simulink model "XfmrProtection_300MVA_Yd1"  (R2023a)
settings: Solver=ode23tb  StartTime=0.0  StopTime=0.30  MaxStep=2e-5  RelTol=1e-5
libraries: spsThreePhaseFaultLib x5, spsThreePhaseSeriesRLCBranchLib x5, spsThreePhaseVIMeasurementLib x4, spsThreePhaseBreakerLib x1, spsGroundLib x1, spsThreePhaseTransformerTwoWindingsLib x1, spsThreePhaseSourceLib x1, spspowerguiLib x1
settings Model: Creator=Abeer  LastModifiedBy=Abeer

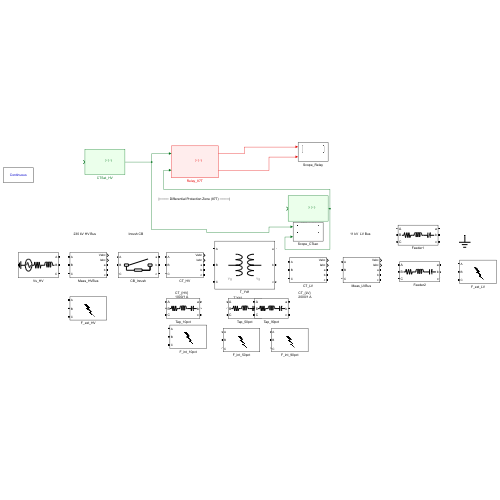
[thumbnail: Simulink's stored preview of the top-level diagram]
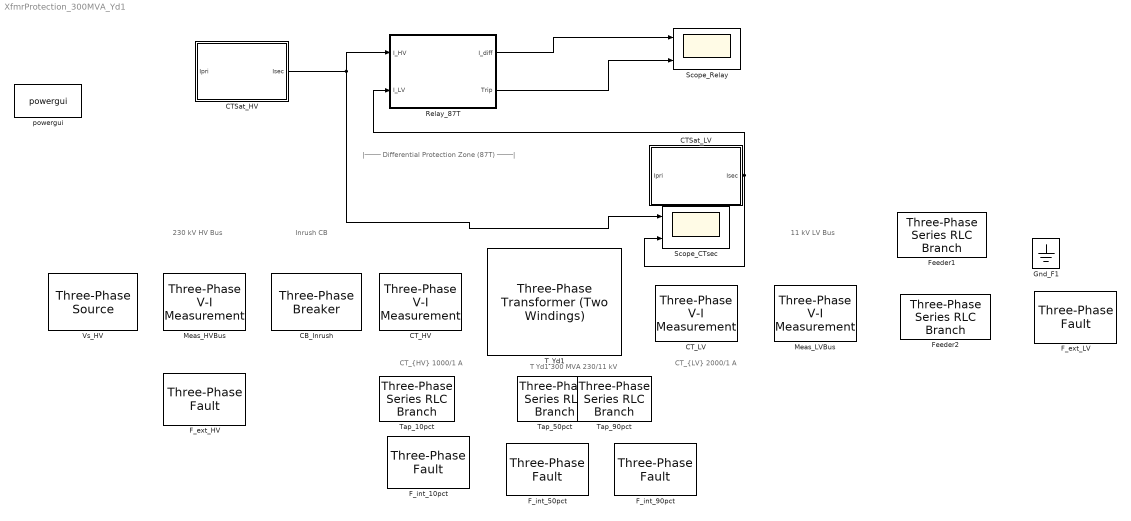
== system XfmrProtection_300MVA_Yd1 ==
  note: 230 kV HV Bus
  note: 11 kV LV Bus
  note: T Yd1
      | 300 MVA
      | 230/11 kV
  note: CT_{HV}
      | 1000/1 A
  note: CT_{LV}
      | 2000/1 A
  note: Inrush CB
  note: |──── Differential Protection Zone (87T) ────|
  CB_Inrush : spsThreePhaseBreakerLib/Three-Phase Breaker  InitialState=open  SwitchA=on  SwitchB=on  SwitchC=on  SwitchTimes="[1/60  5/60]"  External=off  BreakerResistance=0.01  SnubberResistance=1e6  SnubberCapacitance=inf  Measurements=None
  CTSat_HV : Subsystem
      mask Display: color([0 0.45 0.1]);patch([0.08 0.92 0.92 0.08],[0.08 0.08 0.92 0.92],[0.92 1.0 0.92]);text(0.5,0.62,'CTSat_HV','hor','center','FontSize',8,'FontWeight','bold');text(0.5,0.32,'Sat CT','hor','center','FontSize',7);text(0.5,0.15,'1/1000','hor','center','FontSize',7);
  CTSat_LV : Subsystem
      mask Display: color([0 0.45 0.1]);patch([0.08 0.92 0.92 0.08],[0.08 0.08 0.92 0.92],[0.92 1.0 0.92]);text(0.5,0.62,'CTSat_LV','hor','center','FontSize',8,'FontWeight','bold');text(0.5,0.32,'Sat CT','hor','center','FontSize',7);text(0.5,0.15,'1/2000','hor','center','FontSize',7);
  CT_HV : spsThreePhaseVIMeasurementLib/Three-Phase V-I Measurement  VoltageMeasurement=phase-to-ground  SetLabelV=off  LabelV=Vabc  Vpu=off  VpuLL=off  CurrentMeasurement=yes  SetLabelI=off  LabelI=Iabc  Ipu=off  Pbase=100e6  Vbase=500e3  OutputType=Complex  PhasorSimulation=off  PSBequivalent=0
  CT_LV : spsThreePhaseVIMeasurementLib/Three-Phase V-I Measurement  VoltageMeasurement=phase-to-ground  SetLabelV=off  LabelV=Vabc  Vpu=off  VpuLL=off  CurrentMeasurement=yes  SetLabelI=off  LabelI=Iabc  Ipu=off  Pbase=100e6  Vbase=500e3  OutputType=Complex  PhasorSimulation=off  PSBequivalent=0
  F_ext_HV : spsThreePhaseFaultLib/Three-Phase Fault  InitialStates=0  FaultA=on  FaultB=on  FaultC=on  GroundFault=on  SwitchTimes="[1/60  5/60]"  External=off  SwitchStatus=NaN  FaultResistance=0.001  GroundResistance=0.01  SnubberResistance=1e6  SnubberCapacitance=inf  Measurements=None
  F_ext_LV : spsThreePhaseFaultLib/Three-Phase Fault  InitialStates=0  FaultA=on  FaultB=on  FaultC=on  GroundFault=on  SwitchTimes="[1/60  5/60]"  External=off  SwitchStatus=NaN  FaultResistance=0.001  GroundResistance=0.01  SnubberResistance=1e6  SnubberCapacitance=inf  Measurements=None
  F_int_10pct : spsThreePhaseFaultLib/Three-Phase Fault  InitialStates=0  FaultA=on  FaultB=on  FaultC=on  GroundFault=on  SwitchTimes="[1/60  5/60]"  External=off  SwitchStatus=NaN  FaultResistance=0.001  GroundResistance=0.01  SnubberResistance=1e6  SnubberCapacitance=inf  Measurements=None
  F_int_50pct : spsThreePhaseFaultLib/Three-Phase Fault  InitialStates=0  FaultA=on  FaultB=on  FaultC=on  GroundFault=on  SwitchTimes="[1/60  5/60]"  External=off  SwitchStatus=NaN  FaultResistance=0.001  GroundResistance=0.01  SnubberResistance=1e6  SnubberCapacitance=inf  Measurements=None
  F_int_90pct : spsThreePhaseFaultLib/Three-Phase Fault  InitialStates=0  FaultA=on  FaultB=on  FaultC=on  GroundFault=on  SwitchTimes="[1/60  5/60]"  External=off  SwitchStatus=NaN  FaultResistance=0.001  GroundResistance=0.01  SnubberResistance=1e6  SnubberCapacitance=inf  Measurements=None
  Feeder1 : spsThreePhaseSeriesRLCBranchLib/Three-Phase Series RLC Branch  LConnTagsString=A|B|C  RConnTagsString=A|B|C  BranchType=RLC  Resistance=1  Inductance=1e-3  Capacitance=1e-6  Measurements=None
  Feeder2 : spsThreePhaseSeriesRLCBranchLib/Three-Phase Series RLC Branch  LConnTagsString=A|B|C  RConnTagsString=A|B|C  BranchType=RLC  Resistance=1  Inductance=1e-3  Capacitance=1e-6  Measurements=None
  Gnd_F1 : spsGroundLib/Ground  LConnTagsString=a
  Meas_HVBus : spsThreePhaseVIMeasurementLib/Three-Phase V-I Measurement  VoltageMeasurement=phase-to-ground  SetLabelV=off  LabelV=Vabc  Vpu=off  VpuLL=off  CurrentMeasurement=yes  SetLabelI=off  LabelI=Iabc  Ipu=off  Pbase=100e6  Vbase=500e3  OutputType=Complex  PhasorSimulation=off  PSBequivalent=0
  Meas_LVBus : spsThreePhaseVIMeasurementLib/Three-Phase V-I Measurement  VoltageMeasurement=phase-to-ground  SetLabelV=off  LabelV=Vabc  Vpu=off  VpuLL=off  CurrentMeasurement=yes  SetLabelI=off  LabelI=Iabc  Ipu=off  Pbase=100e6  Vbase=500e3  OutputType=Complex  PhasorSimulation=off  PSBequivalent=0
  Relay_87T : Subsystem
      mask Display: color('red');patch([0.05 0.95 0.95 0.05],[0.05 0.05 0.95 0.95],[1 0.93 0.93]);text(0.5,0.60,'87T','hor','center','ver','middle','FontSize',14,'FontWeight','bold');text(0.5,0.20,'Diff Relay','hor','center','FontSize',7);
  Scope_CTsec : Scope  NumInputPorts=2
  Scope_Relay : Scope  NumInputPorts=2
  T_Yd1 : spsThreePhaseTransformerTwoWindingsLib/Three-Phase Transformer (Two Windings)  Winding1Connection=Yg  Winding2Connection=Yg  CoreType=Three single-phase transformers  SetSaturation=off  Hysteresis=off  DataFile='hysteresis'  SetInitialFlux=off  Measurements=None  UNITS=pu  NominalPower=[ 250e6 , 60 ]  Winding1=[ 735e3 , 0.002 , 0.08 ]  Winding2=[ 315e3 , 0.002 , 0.08 ]  Rm=500  Lm=500  L0=0.5  Saturation=[ 0,0 ; 0.0024,1.2 ; 1.0,1.52 ]  InitialFluxes=[ 0.8 , -0.8 , 0.7 ]  BreakLoop=off  DiscreteSolver=Trapezoidal iterative  DataType=off  TransfoNumber=1
  Tap_10pct : spsThreePhaseSeriesRLCBranchLib/Three-Phase Series RLC Branch  LConnTagsString=A|B|C  RConnTagsString=A|B|C  BranchType=RLC  Resistance=1  Inductance=1e-3  Capacitance=1e-6  Measurements=None
  Tap_50pct : spsThreePhaseSeriesRLCBranchLib/Three-Phase Series RLC Branch  LConnTagsString=A|B|C  RConnTagsString=A|B|C  BranchType=RLC  Resistance=1  Inductance=1e-3  Capacitance=1e-6  Measurements=None
  Tap_90pct : spsThreePhaseSeriesRLCBranchLib/Three-Phase Series RLC Branch  LConnTagsString=A|B|C  RConnTagsString=A|B|C  BranchType=RLC  Resistance=1  Inductance=1e-3  Capacitance=1e-6  Measurements=None
  Vs_HV : spsThreePhaseSourceLib/Three-Phase Source  InternalConnection=Yg  VoltagePhases=off  Voltage=25e3  PhaseAngle=0  Voltage_phases=[25e3 25e3 25e3]/sqrt(3)  PhaseAngles_phases=[0 -120 +120]  Frequency=60  NonIdealSource=on  SpecifyImpedance=off  Resistance=0.8929  Inductance=16.58e-3  ShortCircuitLevel=100e6  BaseVoltage=25e3  XRratio=7  BusType=swing  Pref=10e3  Qref=0  Prefabc=[10e3, 10e3, 10e3]  Qrefabc=[0, 0, 0]  Qmin=-inf  Qmax=inf
  powergui : spspowerguiLib/powergui  Priority=1  SimulationMode=Continuous  SampleTime=50e-6  frequency=60  Iterations=50  frequencyindice=60  Pbase=100e6  ErrMax=1e-4  UnitsV=kV  UnitsW=MW  buscounter=0  FunctionMessages=off  echomessages=off  EnableUseOfTLC=off  CurrentSourceSwitches=off  DisableSnubberDevices=off  DisableRonSwitches=off  DisableVfSwitches=off  DisplayEquations=off  AutomaticDiscreteSolvers=off  SolverType=Tustin/Backward Euler (TBE)  Interpol=off  ExternalGateDelay=off  methode=off  Ts=100  x0status=blocks  SPID=on  SwTol=0  HookPort=off  NonlinearTolerance=1e-4  nMaxIteration=100  ContinueOnMaxIteration=off  RestoreLinks=warning  ResistiveCurrentMeasurement=off  Frange=[0:2:500]  Ylog=off  Xlog=on  ShowGrid=off  save=off  variable=ZData  structure=0  ZoomFFT=off  StartTime=0.0  cycles=1  DisplayStyle=1  fundamental=60  FreqAxis=off  MaxFrequency=1000  frequencyindicesteady=1  RmsSteady=1  display=off
  wires:
  CTSat_HV/1(Isec) -> Scope_CTsec/1, Relay_87T/1(I_HV)
  CTSat_LV/1(Isec) -> Relay_87T/2(I_LV), Scope_CTsec/2
  Relay_87T/1(I_diff) -> Scope_Relay/1
  Relay_87T/2(Trip) -> Scope_Relay/2

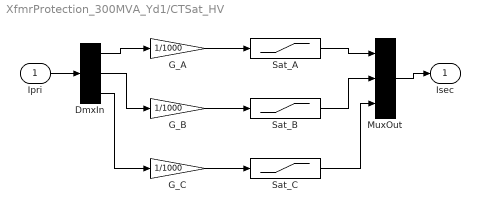
== system XfmrProtection_300MVA_Yd1/CTSat_HV ==
  Ipri : Inport
  DmxIn : Demux  Outputs=3
  G_A : Gain  Gain=1/1000
  G_B : Gain  Gain=1/1000
  G_C : Gain  Gain=1/1000
  MuxOut : Mux  Inputs=3
  Sat_A : Saturate  UpperLimit=1.0  LowerLimit=-1.0
  Sat_B : Saturate  UpperLimit=1.0  LowerLimit=-1.0
  Sat_C : Saturate  UpperLimit=1.0  LowerLimit=-1.0
  Isec : Outport
  wires:
  Ipri/1 -> DmxIn/1
  DmxIn/1 -> G_A/1
  G_A/1 -> Sat_A/1
  Sat_A/1 -> MuxOut/1
  DmxIn/2 -> G_B/1
  G_B/1 -> Sat_B/1
  Sat_B/1 -> MuxOut/2
  DmxIn/3 -> G_C/1
  G_C/1 -> Sat_C/1
  Sat_C/1 -> MuxOut/3
  MuxOut/1 -> Isec/1

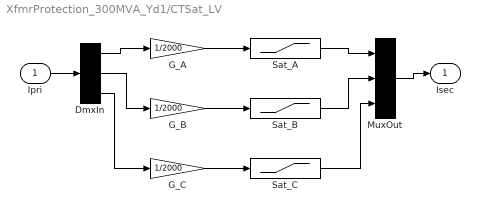
== system XfmrProtection_300MVA_Yd1/CTSat_LV ==
  Ipri : Inport
  DmxIn : Demux  Outputs=3
  G_A : Gain  Gain=1/2000
  G_B : Gain  Gain=1/2000
  G_C : Gain  Gain=1/2000
  MuxOut : Mux  Inputs=3
  Sat_A : Saturate  UpperLimit=1.0  LowerLimit=-1.0
  Sat_B : Saturate  UpperLimit=1.0  LowerLimit=-1.0
  Sat_C : Saturate  UpperLimit=1.0  LowerLimit=-1.0
  Isec : Outport
  wires:
  Ipri/1 -> DmxIn/1
  DmxIn/1 -> G_A/1
  G_A/1 -> Sat_A/1
  Sat_A/1 -> MuxOut/1
  DmxIn/2 -> G_B/1
  G_B/1 -> Sat_B/1
  Sat_B/1 -> MuxOut/2
  DmxIn/3 -> G_C/1
  G_C/1 -> Sat_C/1
  Sat_C/1 -> MuxOut/3
  MuxOut/1 -> Isec/1

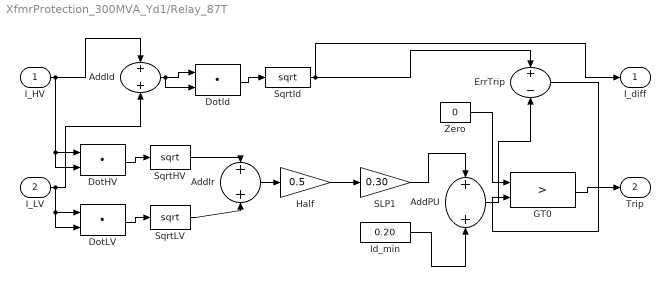
== system XfmrProtection_300MVA_Yd1/Relay_87T ==
  I_HV : Inport
  I_LV : Inport  Port=2
  AddId : Sum
  AddIr : Sum
  AddPU : Sum
  DotHV : DotProduct  OutDataTypeStr=Inherit: Inherit via internal rule
  DotId : DotProduct  OutDataTypeStr=Inherit: Inherit via internal rule
  DotLV : DotProduct  OutDataTypeStr=Inherit: Inherit via internal rule
  ErrTrip : Sum  Inputs=+-
  GT0 : RelationalOperator  Operator=>  OutDataTypeStr=boolean  RndMeth=Simplest  InputSameDT=off
  Half : Gain  Gain=0.5
  Id_min : Constant  Value=0.20
  SLP1 : Gain  Gain=0.30
  SqrtHV : Sqrt
  SqrtId : Sqrt
  SqrtLV : Sqrt
  Zero : Constant  Value=0
  I_diff : Outport
  Trip : Outport  Port=2
  wires:
  I_HV/1 -> DotHV/1, DotHV/2, AddId/1
  I_LV/1 -> DotLV/1, DotLV/2, AddId/2
  AddId/1 -> DotId/1, DotId/2
  DotId/1 -> SqrtId/1
  DotHV/1 -> SqrtHV/1
  DotLV/1 -> SqrtLV/1
  SqrtHV/1 -> AddIr/1
  SqrtLV/1 -> AddIr/2
  AddIr/1 -> Half/1
  Half/1 -> SLP1/1
  SLP1/1 -> AddPU/1
  Id_min/1 -> AddPU/2
  SqrtId/1 -> ErrTrip/1, I_diff/1
  AddPU/1 -> ErrTrip/2
  Zero/1 -> GT0/1
  ErrTrip/1 -> GT0/2
  GT0/1 -> Trip/1
